simulink model "smc_tracking"  (R2024b)
settings: Solver=FixedStepAuto  StartTime=0.0  StopTime=10  FixedStep=1e-5  MaxStep=1e-4  RelTol=1e-6  AbsTol=1e-4
values from neighbouring files (symbols this model uses):
  Ampdes = 2.2    [Chapter2.m]    (also in FBL.m; LinearControl.m; SlidingMode.m; control.m)
  Biasdes = 3.3    [Chapter2.m]    (also in FBL.m; LinearControl.m; SlidingMode.m; control.m)
  Freqdes = 2*pi/6    (= 1.0471975512)    [Chapter2.m]    (also in FBL.m; LinearControl.m; SlidingMode.m; control.m)
  Phasedes = 3*pi/2    (= 4.71238898038)    [Chapter2.m]    (also in FBL.m; LinearControl.m; SlidingMode.m; control.m)
  x_0 = [1; 7; 7]    [Chapter2.m]    (also in FBL.m; LinearControl.m; SlidingMode.m; control.m)
settings Model: Creator=User  LastModifiedBy=robyr

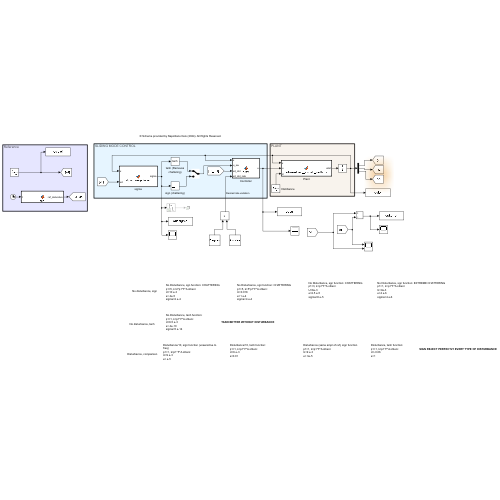
[thumbnail: Simulink's stored preview of the top-level diagram]
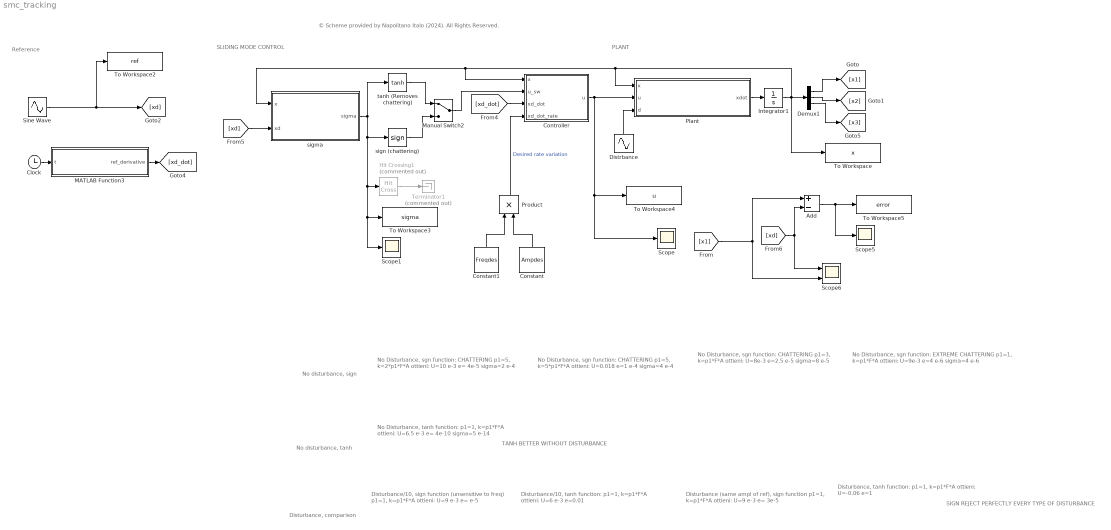
== system smc_tracking ==
  note: No disturbance, sign
  note: TANH BETTER WITHOUT DISTURBANCE
  note: SIGN REJECT PERFECTLY EVERY TYPE OF DISTURBANCE
  note: PLANT
  note: Reference
  note: SLIDING MODE CONTROL
  note: © Scheme provided by Napolitano Italo (2024). All Rights Reserved.
  note: No Disturbance, sgn function: CHATTERING
      | p1=5, k=2*p1*F*A ottieni:
      | U=10 e-3
      | e= 4e-5
      | sigma=2 e-4
  note: No Disturbance, sgn function: CHATTERING
      | p1=5, k=5*p1*F*A ottieni:
      | U=0.018
      | e=1 e-4
      | sigma=4 e-4
  note: No Disturbance, sgn function: CHATTERING
      | p1=3, k=p1*F*A ottieni:
      | U=8e-3
      | e=2.5 e-5
      | sigma=8 e-5
  note: No Disturbance, sgn function: EXTREME CHATTERING
      | p1=1, k=p1*F*A ottieni:
      | U=9e-3
      | e=4 e-6
      | sigma=4 e-6
  note: No Disturbance, tanh function:
      | p1=1, k=p1*F*A ottieni:
      | U=6.5 e-3
      | e= 4e-10
      | sigma=5 e-14
  note: Disturbance/10, sign function (unsensitive to freq)
      | p1=1, k=p1*F*A ottieni:
      | U=9 e-3
      | e= e-5
  note: Disturbance/10, tanh function:
      | p1=1, k=p1*F*A ottieni:
      | U=6 e-3
      | e=0.01
  note: Disturbance (same ampl of ref), sign function
      | p1=1, k=p1*F*A ottieni:
      | U=9 e-3
      | e= 3e-5
  note: Disturbance, tanh function:
      | p1=1, k=p1*F*A ottieni:
      | U=-0.06
      | e=1
  note: No disturbance, tanh
  note: Disturbance, comparison
  Add : Sum  Inputs=+-
  Clock : Clock
  Constant : Constant  Value=Ampdes
  Constant1 : Constant  Value=Freqdes
  Controller : MATLAB Function  TreatAsAtomicUnit=on
  Demux1 : Demux  Outputs=3
  Distrbance : Sin  Amplitude=Ampdes  Frequency=Freqdes  Phase=Phasedes  SampleTime=0
  Hit Crossing1 : HitCross  Commented=on
  Integrator1 : Integrator  InitialCondition=x_0
  MATLAB Function3 : MATLAB Function  TreatAsAtomicUnit=on
  Manual Switch2 : ManualSwitch
  Plant : MATLAB Function  TreatAsAtomicUnit=on
  Product : Product
  Scope : Scope
  Scope1 : Scope
  Scope5 : Scope
  Scope6 : Scope  NumInputPorts=2
  Sine Wave : Sin  Amplitude=Ampdes  Bias=Biasdes  Frequency=Freqdes  Phase=Phasedes  SampleTime=0
  Terminator1 : Terminator  Commented=on
  To Workspace : ToWorkspace  VariableName=x  SaveFormat=Timeseries  SampleTime=-1
  To Workspace2 : ToWorkspace  VariableName=ref  SaveFormat=Timeseries  SampleTime=-1
  To Workspace3 : ToWorkspace  VariableName=sigma  SaveFormat=Timeseries  SampleTime=-1
  To Workspace4 : ToWorkspace  VariableName=u  SaveFormat=Timeseries  SampleTime=-1
  To Workspace5 : ToWorkspace  VariableName=error  SaveFormat=Timeseries  SampleTime=-1
  sigma : MATLAB Function  TreatAsAtomicUnit=on
  sign (chattering) : Signum
  tanh (Removes chattering) : Trigonometry  Operator=tanh
  wires:
  Controller/1(u) -> Plant/2(u), To Workspace4/1, Scope/1
  Plant/1(xdot) -> Integrator1/1
  Integrator1/1 -> To Workspace/1, Demux1/1, sigma/1(x), Controller/1(x), Plant/1(x)
  Manual Switch2/1 -> Controller/2(u_sw)
  sigma/1(sigma) -> tanh (Removes chattering)/1, Scope1/1, To Workspace3/1, Hit Crossing1/1, sign (chattering)/1
  sign (chattering)/1 -> Manual Switch2/2
  tanh (Removes chattering)/1 -> Manual Switch2/1
  Sine Wave/1 -> To Workspace2/1, [xd]
  Hit Crossing1/1 -> Terminator1/1
  Add/1 -> To Workspace5/1, Scope5/1
  Demux1/1 -> [x1]
  Demux1/2 -> [x2]
  [x1] -> Scope6/2, Add/1
  [xd_dot] -> Controller/3(xd_dot)
  [xd] -> sigma/2(xd)
  Demux1/3 -> [x3]
  [xd] -> Scope6/1, Add/2
  Constant/1 -> Product/2
  Constant1/1 -> Product/1
  Product/1 -> Controller/4(xd_dot_rate)  "Desired rate variation"
  Clock/1 -> MATLAB Function3/1(t)
  MATLAB Function3/1(ref_derivative) -> [xd_dot]
  Distrbance/1 -> Plant/3(d)

== matlab function smc_tracking/MATLAB Function3 ==
  data: t input; ref_derivative output
function ref_derivative = fcn(t)

Ampdes=2.2 ;
Freqdes= 2*pi/6; 
Phasedes= 3*pi/2;


ref_derivative = Ampdes * Freqdes * cos(Freqdes * t + Phasedes);

== matlab function smc_tracking/Plant ==
  data: x input; u input; xdot output; d input
function xdot = adimensional_goodwin_oscillator(x,u,d)
b=0.1;
a=b^-3;
n=9;

xdot = [-x(1)+a/(1+x(3)^n) + a*u + d;...
        -x(2)+x(1);...
        -x(3)+ x(2);];

== matlab function smc_tracking/Controller ==
  data: x input; u output; u_sw input; xd_dot input; xd_dot_rate input
function u = SMC(x, u_sw, xd_dot, xd_dot_rate)



%Sys param
b=0.1;
a=b^-3;
n=9;

%Control param
p1=1; %What? High value imply bad tracking?
%p2=1;
k=p1*xd_dot_rate;
%k=3;
%Computed analitically with Lie Derivative
u_eq =  (x(1) - a/(1 + x(3)^n))/a ;
u_sw = - k/(a*p1) * u_sw;
u_ff= xd_dot/a/p1;
u = u_eq + u_sw + u_ff;

== matlab function smc_tracking/sigma ==
  data: x input; sigma output; xd input
function sigma = sigma_computation(x,xd)
%Tracking for x1 only:

p1=1;
%p2=1;
%I Cant add there the tracking term, i havent x1dot -> go add FF in u
sigma = p1*(x(1)-xd);

end
